simulink model "Draw_Graph_Flex_Vol_SIMULINK"  (R2023a)
settings: Solver=FixedStepAuto  StartTime=0.0  StopTime=inf  FixedStep=0.01  RelTol=1e-3  EnableMultiTasking=on
libraries: dspfdesign x2, arduinolib x1
settings Model: ExtModeTrigDuration=2  Creator=PHUC  LastModifiedBy=PHUC
settings SolverCC: AutoInsertRateTranBlk=on
settings OptimizationCC: EnhancedBackFolding=on  PassReuseOutputArgsAs=Individual arguments  ZeroExternalMemoryAtStartup=off  ZeroInternalMemoryAtStartup=off  MaxStackSize=64  OptimizeBlockOrder=speed  DifferentSizesBufferReuse=on  OptimizationCustomize=off  EfficientTunableParamExpr=on
settings DebuggingCC: ParameterTunabilityLossMsg=error
settings HardwareCC: ProdBitPerInt=16  ProdBitPerPointer=16  ProdBitPerSizeT=16  ProdBitPerPtrDiffT=16  ProdLargestAtomicFloat=None  ProdWordSize=8  ProdHWDeviceType=Atmel->AVR
settings SFSimCC: MATLABDynamicMemAlloc=off
settings RTWCC: Description=Embedded Coder  SystemTargetFile=ert.tlc  HardwareBoard=Arduino Mega 2560  TemplateMakefile=ert_default_tmf  Toolchain=Arduino AVR  BuildConfiguration=Faster Runs
settings CodeAppCC: ForceParamTrailComments=on  IgnoreCustomStorageClasses=off  OperatorAnnotations=on  SimulinkDataObjDesc=on  SFDataObjDesc=on  InsertBlockDesc=on
settings ERTTargetCC: SupportContinuousTime=on  SupportVariableSizeSignals=on  ExtModeTransport=3  ExtModeStaticAlloc=on  ExtModeAutomaticAllocSize=off  ExtModeStaticAllocSize=2048  ExtModeMexFile=ext_xcp  ExtModeIntrfLevel=Level2 - Open

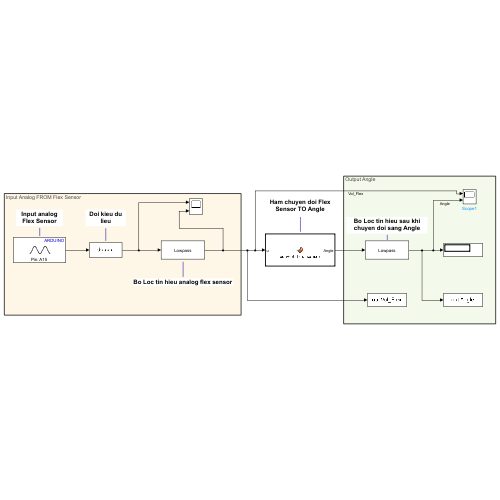
[thumbnail: Simulink's stored preview of the top-level diagram]
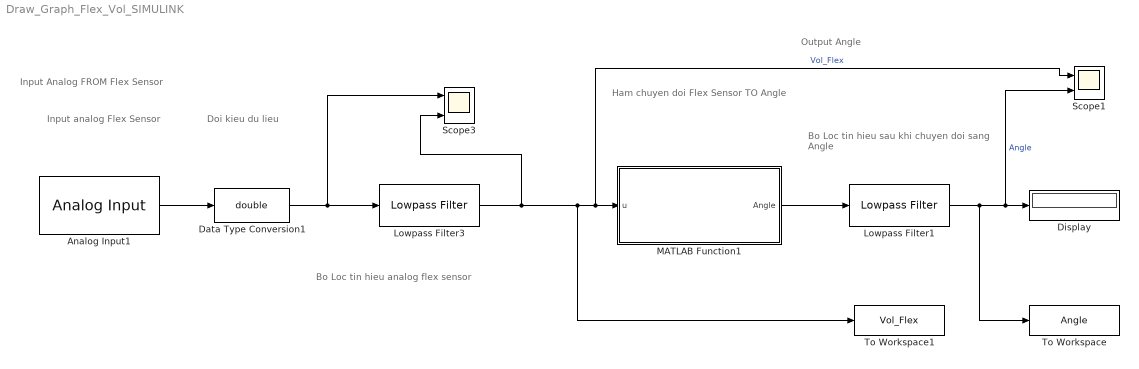
== system Draw_Graph_Flex_Vol_SIMULINK ==
  note: Output Angle
  note: Doi kieu du lieu
  note: Bo Loc tin hieu analog flex sensor
  note: Input Analog FROM Flex Sensor
  note: Input analog Flex Sensor
  note: Ham chuyen doi Flex Sensor TO Angle
  note: Bo Loc tin hieu sau khi chuyen doi sang Angle
  Analog Input1 : arduinolib/Analog Input  pinNumber=15  ReadResultsOnly=off  ConversionTriggerSource=Software  ExternalTriggerType=uint32( 0 )  OutputDataType=uint16  EnableConversionCompleteNotify=off  EnableOuputStatus=off  SampleTime=-1  blockPlatform=arduino
  Data Type Conversion1 : DataTypeConversion  OutDataTypeStr=double  SaturateOnIntegerOverflow=off  RndMeth=Floor
  Display : Display
  Lowpass Filter1 : dspfdesign/Lowpass Filter  FilterType=FIR  DesignForMinimumOrder=off  FilterOrder=20  PassbandFrequency=0.01e2  StopbandFrequency=12e3  PassbandRipple=0.001  StopbandAttenuation=50  SampleRateMode=Specify on dialog  SampleRate=44100  SimulateUsing=Interpreted execution  roundingMode=Floor  coeffsDataTypeStr=fixdt(1,16)
  Lowpass Filter3 : dspfdesign/Lowpass Filter  FilterType=FIR  DesignForMinimumOrder=off  FilterOrder=20  PassbandFrequency=0.1e3  StopbandFrequency=12e3  PassbandRipple=0.001  StopbandAttenuation=50  SampleRateMode=Specify on dialog  SampleRate=44100  SimulateUsing=Interpreted execution  roundingMode=Floor  coeffsDataTypeStr=fixdt(1,16)
  MATLAB Function1 : MATLAB Function  TreatAsAtomicUnit=on
  Scope1 : Scope  NumInputPorts=2
  Scope3 : Scope  NumInputPorts=2
  To Workspace : ToWorkspace  VariableName=Angle  SaveFormat=Timeseries  SampleTime=-1
  To Workspace1 : ToWorkspace  VariableName=Vol_Flex  SaveFormat=Timeseries  SampleTime=-1
  wires:
  Analog Input1/1 -> Data Type Conversion1/1
  Data Type Conversion1/1 -> Lowpass Filter3/1, Scope3/1
  Lowpass Filter3/1 -> MATLAB Function1/1(u), Scope1/1, To Workspace1/1, Scope3/2  "Vol_Flex"
  MATLAB Function1/1(Angle) -> Lowpass Filter1/1
  Lowpass Filter1/1 -> Display/1, Scope1/2, To Workspace/1  "Angle"

== matlab function Draw_Graph_Flex_Vol_SIMULINK/MATLAB Function1 ==
  data: u input; Angle output
function Angle  = convert_flex_sensor(u)

VCC = 4.98;
R_DIV = 47500.0;
STRAIGHT_RESISTANCE = 24000.0;
BEND_RESISTANCE = 30000.0;


flexV = u * VCC / 1023.0;
flexR = R_DIV * (VCC / flexV - 1.0);

Angle = (((flexR - STRAIGHT_RESISTANCE)/(BEND_RESISTANCE - STRAIGHT_RESISTANCE))*90.0);
